simulink model "q1"  (R2023a)
settings: Solver=VariableStepAuto  StartTime=0.0  StopTime=10.0  RelTol=1e-3
settings Model: Creator=phateme  LastModifiedBy=phateme

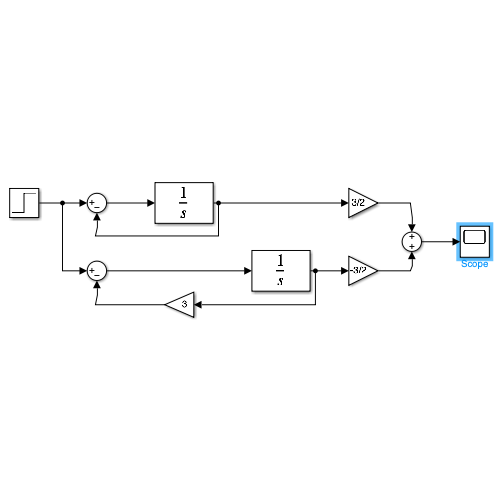
[thumbnail: Simulink's stored preview of the top-level diagram]
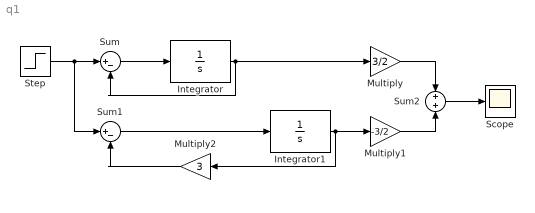
== system q1 ==
  Integrator : Integrator
  Integrator1 : Integrator
  Multiply : Gain  Gain=3/2
  Multiply1 : Gain  Gain=-3/2
  Multiply2 : Gain  Gain=3
  Scope : Scope
  Step : Step  Time=0  SampleTime=0
  Sum : Sum  Inputs=|+-
  Sum1 : Sum  Inputs=|+-
  Sum2 : Sum
  wires:
  Multiply1/1 -> Sum2/2
  Sum2/1 -> Scope/1
  Multiply/1 -> Sum2/1
  Integrator/1 -> Multiply/1, Sum/2
  Multiply2/1 -> Sum1/2
  Integrator1/1 -> Multiply1/1, Multiply2/1
  Step/1 -> Sum1/1, Sum/1
  Sum1/1 -> Integrator1/1
  Sum/1 -> Integrator/1
